simulink model "CorrecteurSimulee"  (R2020a)
settings: Solver=FixedStepAuto  StartTime=0.0  StopTime=30  FixedStep=Te  RelTol=1e-3
undefined symbols (not defined in the file or in its folder): GzMain, PI1
settings Model: Creator=garnica-aza  LastModifiedBy=garnica-aza

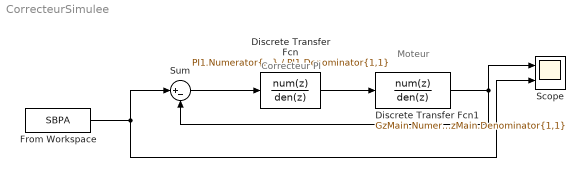
== system CorrecteurSimulee ==
  note: Moteur
  note: Correcteur PI
  Discrete Transfer Fcn : DiscreteTransferFcn  Numerator=PI1.Numerator{1,1}  Denominator=PI1.Denominator{1,1}
  Discrete Transfer Fcn1 : DiscreteTransferFcn  Numerator=GzMain.Numerator{1,1}  Denominator=GzMain.Denominator{1,1}
  From Workspace : FromWorkspace  VariableName=SBPA
  Scope : Scope  NumInputPorts=2
  Sum : Sum  Inputs=|+-
  wires:
  Sum/1 -> Discrete Transfer Fcn/1
  Discrete Transfer Fcn/1 -> Discrete Transfer Fcn1/1
  Discrete Transfer Fcn1/1 -> Scope/1, Sum/2
  From Workspace/1 -> Sum/1, Scope/2
